simulink model "NLGuidance"  (R2016a)
settings: Solver=ode3  StartTime=0.0  StopTime=10.0  FixedStep=.02  RelTol=1e-3
model workspace (MAT data in the model file):
  F = [0.0104799567177; 0.0105274136759; 0.00258730184958; 0.00112291450915; 0.0065543125439; 0]
  N = 51
  S1 = [2.42464759278 -2.49697623385 -0.253883104432 -3.312058597 3.28063521535 2.42464759278 -2.49697623385 -0.253883104432 -3.312058597 3.28063521535 2.42464759278 -2.49697623385 ... (7515 elements, 5x1503)]
  S2 = [-47.5753524072 -52.4969762338 -50.2538831044 -53.312058597 -46.7193647847 -53.1933464928 -58.0206597562 -53.298625948 -53.0732596071 -45.5277132009 -58.8093605499 -63.5421671216 ... (7515 elements, 5x1503)]
  S3 = [-5.62481372887 -5.52769980874 -3.05143765206 0.237149289911 1.1849461568 -5.61799408553 -5.52368352234 -3.04474284358 0.238798989919 1.19165158379 -5.61601405716 -5.52150736543 ... (7515 elements, 5x1503)]
  S4 = [0 0 0 0 0 0 0 0 0 0 0 0 ... (7515 elements, 5x1503)]
  Vt = [0 0 0 0 0 0 0 0 0 0 0 0 ... (1503 elements, 501x3)]
  Vv = [1.1849461568 1.19165158379 1.19363427504 1.1947051518 1.20742767257 1.21177592763 1.21717805586 1.22205358332 1.22753574851 1.22892415591 1.22911717004 1.25058652202 ... (1503 elements, 501x3)]
  Vvmag = [6.45855507903 6.44973720458 6.44685088198 6.4408859639 6.4366826743 6.42659096353 6.42411891458 6.41278379056 6.40944425236 6.4051659263 6.38964384833 6.38667032718 ... (501 elements, 501x1)]
  X = [2.42464759278 -2.49697623385 -0.253883104432 -3.312058597 3.28063521535 -3.6978315289 -3.58806283515 -3.26410626081 1.58732884776 1.68742830515 1.89810778603 -3.58806283515 ... (72 elements, 6x12)]
  Xap1 = [3.53742766553 3.54841812521 3.55649436401 3.56301032299 3.56900127601 3.57285766144 3.57579889741 3.57816116305 3.57954580685 3.57954139291 3.5792899619 3.58161806007 ... (1503 elements, 501x3)]
  Xap2 = [3.00894026262 2.99947384008 2.99278206158 2.98751350515 2.98264302934 2.97978827516 2.97774180284 2.97617755456 2.97550435147 2.97614326838 2.97696071264 2.97513994677 ... (1503 elements, 501x3)]
  Xr = [10 11.2284720857 12.4539847001 13.6735561742 14.8879723634 16.0937793652 17.2959786101 18.4820399899 19.6645679603 20.8393619799 21.9947001613 23.1446286766 ... (1503 elements, 501x3)]
  Xrmag = [15.65732221 23.8105907731 30.9856356907 38.4540834067 46.0738528973 53.7662892745 61.5065103501 69.2725920166 77.0607192366 84.8582850512 92.6527324163 100.450411961 ... (501 elements, 501x1)]
  Xtarg = [3.28063521535 3.28063521535 3.28063521535 3.28063521535 3.28063521535 3.28063521535 3.28063521535 3.28063521535 3.28063521535 3.28063521535 3.28063521535 3.28063521535 ... (1503 elements, 501x3)]
  Xv = [-46.7193647847 -45.5277132009 -44.3340789258 -43.139373774 -41.9319461015 -40.7201701738 -39.502992118 -38.2809385346 -37.0534027861 -35.8244786302 -34.5953614602 -33.3447749382 ... (1503 elements, 501x3)]
  ans = [0  0  0; 2  2  2; 4  4  4]
  MCOS : class17 (value not decoded)
  cmd1 = []
  cmd2 = []
  count = 136
  curPath = '/Users/khouloud.gaaloul/Documents/Projects/QRA-Search/Problems/SimulinkTesting'
  MCOS : class17 (value not decoded)
  MCOS : class17 (value not decoded)
  MCOS : class17 (value not decoded)
  MCOS : class17 (value not decoded)
  d = 10
  dev = [0.998411888767 0.99782484185 0.997422855714 0.997059153759 0.99673360256 0.996441028681 0.996174188817 0.995929724086 0.995704685947 0.995496539497 0.995301805204 0.995118534567 ... (501 elements, 501x1)]
  diff = [-0.0110961446926 -0.0111456874882 -0.0111717248678 -0.0112203324043 -0.0112177067868 -0.0112470382447 -0.0112585651595 -0.0112536842015 -0.0112567920009 -0.0112598719834 -0.0112758132864 -0.011238461177 ... (500 elements, 500x1)]
  MCOS : class17 (value not decoded)
  MCOS : class17 (value not decoded)
  MCOS : class17 (value not decoded)
  handle : class17 (value not decoded)
  i = 26
  inputSize = 6
  j = 3
  list : struct (value not decoded)
  m = [-0.999723895919 -0.999364400237 -0.991672916331 -0.981758345493 -0.98121871348 -0.980992634152 -0.979214833695 -0.97816820181 -0.975813767607 -0.973821424379 -0.973796463479 -0.972935922229 ... (3006 elements, 1002x3)]
  modelpath = '/Users/khouloud.gaaloul/Documents/Projects/QRA-Search/SimulinkModels/4_nlguide/'
  mt = [0.997620134247 0.997296649802 0.994217918569 0.993324313281 0.991703646703 0.985900322398 0.985631450718 0.976402580538 0.973784078633 0.970318825583 0.969896216991 0.965968068121 ... (1503 elements, 501x3)]
  mv = [-0.993370609414 -0.990984924743 -0.989879999798 -0.982454455416 -0.979488128766 -0.978091228792 -0.976254482971 -0.973907633905 -0.96148789861 -0.959724271782 -0.942427931753 -0.941335472094 ... (1503 elements, 501x3)]
  n = 6
  nbrInputs = 4
  nbrTimeSteps = 501
  r2 = 1000000
  s = 4
  MCOS : class17 (value not decoded)
  sumOut = 1.13428583934e-06
  sumVl = 16.4352757808
  t = 501
  var : struct (value not decoded)
  varout : struct (value not decoded)
  x = [2.7049904163 8.31847210292 14.0416550116 19.9218605512 25.7958831948 31.6629046774 37.5137196427 43.3342242648 49.1594101201 54.9752404562 60.7952146721 66.6155429658 ... (501 elements, 501x1)]
  xo = [3.00894026262 2.99947384008 2.99278206158 2.98751350515 2.98264302934 2.97978827516 2.97774180284 2.97617755456 2.97550435147 2.97614326838 2.97696071264 2.97513994677 ... (501 elements, 501x1)]
  xt = [3.28063521535 3.28063521535 3.28063521535 3.28063521535 3.28063521535 3.28063521535 3.28063521535 3.28063521535 3.28063521535 3.28063521535 3.28063521535 3.28063521535 ... (501 elements, 501x1)]
  xv = [-46.7193647847 -45.5277132009 -44.3340789258 -43.139373774 -41.9319461015 -40.7201701738 -39.502992118 -38.2809385346 -37.0534027861 -35.8244786302 -34.5953614602 -33.3447749382 ... (501 elements, 501x1)]
  y = [3.6883959876 9.17834089576 14.9294898906 19.9030920073 24.7285315288 29.5033134454 34.2547577046 38.9972499457 43.7096979702 48.4166380479 53.1197368616 57.8142423866 ... (501 elements, 501x1)]
  yo = [2.64835074056 2.63493178346 2.62207989272 2.61010927833 2.59912240045 2.58878484686 2.57921418375 2.57035768583 2.56215199533 2.55453681534 2.54751560237 2.54111946622 ... (501 elements, 501x1)]
  yout = [3.00894026262 2.99947384008 2.99278206158 2.98751350515 2.98264302934 2.97978827516 2.97774180284 2.97617755456 2.97550435147 2.97614326838 2.97696071264 2.97513994677 ... (1503 elements, 501x3)]
  yt = [1.89810778603 1.89810778603 1.89810778603 1.89810778603 1.89810778603 1.89810778603 1.89810778603 1.89810778603 1.89810778603 1.89810778603 1.89810778603 1.89810778603 ... (501 elements, 501x1)]
  yv = [-48.101892214 -52.3846332875 -56.663611085 -60.93703548 -65.20593249 -69.4668713892 -73.7274049649 -77.9871267457 -82.2407780144 -86.4920761433 -90.7431651505 -94.9853167819 ... (501 elements, 501x1)]
  z = [4.49604856588 6.72999883369 12.0965927953 17.1688972661 22.1258781778 27.0326381497 31.9068218628 36.7791547029 41.639146818 46.4962544595 51.3440742559 56.1827474075 ... (501 elements, 501x1)]
  zo = [4.92497802224 4.93706839336 4.94912096266 4.96029006041 4.97012356487 4.97983400233 4.98881546471 4.99704254051 5.00481819698 5.01242680713 5.01939367699 5.02450802519 ... (501 elements, 501x1)]
  zt = [4.32221989343 4.32221989343 4.32221989343 4.32221989343 4.32221989343 4.32221989343 4.32221989343 4.32221989343 4.32221989343 4.32221989343 4.32221989343 4.32221989343 ... (501 elements, 501x1)]
  zv = [45.6777801066 48.680795879 51.6837683233 54.6803231469 57.6757020576 60.666276224 63.6537597154 66.6335569064 69.6091973174 72.5839099026 75.5526555129 78.520090746 ... (501 elements, 501x1)]
(part 2 of 2)

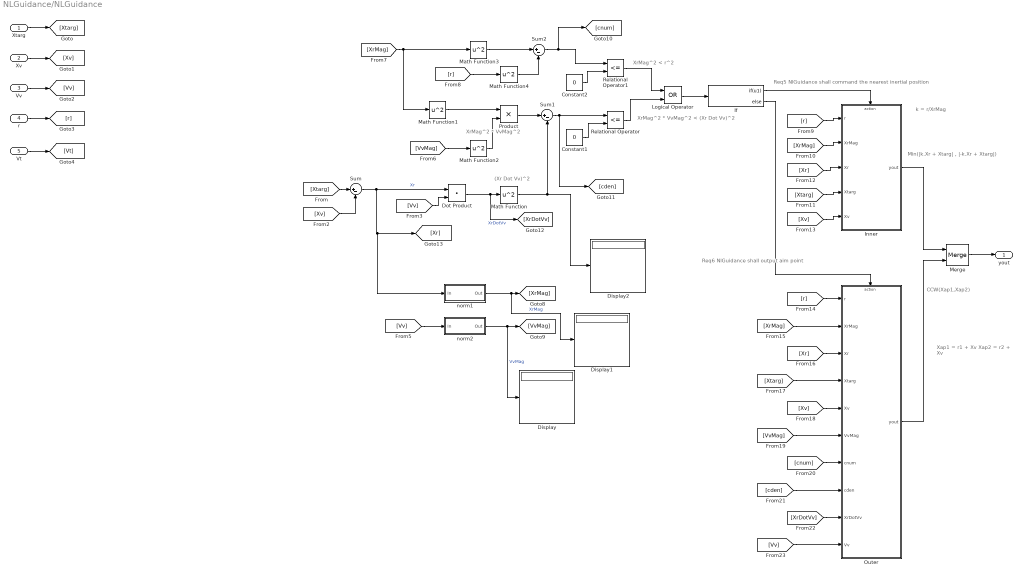
== system NLGuidance/NLGuidance ==
  note: XrMag^2 < r^2
  note: Req5 NlGuidance shall command the nearest inertial position
  note: XrMag^2 * VvMag^2
  note: (Xr Dot Vv)^2
  note: XrMag^2 * VvMag^2 < (Xr Dot Vv)^2
  note: k = r/XrMag
  note: Min(|k.Xr + Xtarg| , |-k.Xr + Xtarg|)
  note: Xap1 = r1 + Xv
      | Xap2 = r2 + Xv
  note: CCW(Xap1,Xap2)
  note: Req6 NlGuidance shall output aim point
  Xtarg : Inport
  Xv : Inport  Port=2
  Vv : Inport  Port=3
  r : Inport  Port=4
  Vt : Inport  Port=5
  Constant1 : Constant  Value=0
  Constant2 : Constant  Value=0
  Display : Display
  Display1 : Display
  Display2 : Display
  Dot Product : DotProduct  InputSameDT=on  OutDataTypeStr=Inherit: Inherit via internal rule
  If : If  IfExpression=u1
  Inner : Subsystem
  Logical Operator : Logic  Operator=OR  AllPortsSameDT=off  OutDataTypeStr=boolean
  Math Function{,1..4} (5 alike) : Math  Operator=square  SaturateOnIntegerOverflow=on
  Merge : Merge
  Outer : Subsystem
  Product : Product  RndMeth=Zero
  Relational Operator : RelationalOperator  Operator=<=  OutDataTypeStr=boolean
  Relational Operator1 : RelationalOperator  Operator=<=  OutDataTypeStr=boolean
  Sum : Sum  Inputs=|+-
  Sum1 : Sum  Inputs=|+-
  Sum2 : Sum  Inputs=|+-
  norm1 : Subsystem
  norm2 : Subsystem
  yout : Outport
  wires:
  Xtarg/1 -> [Xtarg]
  Xv/1 -> [Xv]
  Vv/1 -> [Vv]
  r/1 -> [r]
  Vt/1 -> [Vt]
  [Xtarg] -> Sum/1
  [Xv] -> Sum/2
  Sum/1 -> norm1/1(In), [Xr], Dot Product/1  "Xr"
  [Vv] -> Dot Product/2
  Dot Product/1 -> [XrDotVv], Math Function/1  "XrDotVv"
  norm1/1(Out) -> Display1/1, [XrMag]  "XrMag"
  [Vv] -> norm2/1(In)
  norm2/1(Out) -> Display/1, [VvMag]  "VvMag"
  Math Function/1 -> Display2/1, Sum1/2
  [VvMag] -> Math Function2/1
  Math Function1/1 -> Product/1
  Math Function2/1 -> Product/2
  Product/1 -> Sum1/1
  Sum1/1 -> [cden], Relational Operator/1
  Constant1/1 -> Relational Operator/2
  Relational Operator/1 -> Logical Operator/2
  Sum2/1 -> [cnum], Relational Operator1/1
  Constant2/1 -> Relational Operator1/2
  Relational Operator1/1 -> Logical Operator/1
  Math Function3/1 -> Sum2/1
  [XrMag] -> Math Function1/1, Math Function3/1
  Math Function4/1 -> Sum2/2
  [r] -> Math Function4/1
  [r] -> Inner/1(r)
  [XrMag] -> Inner/2(XrMag)
  Logical Operator/1 -> If/1
  [Xtarg] -> Inner/4(Xtarg)
  [Xr] -> Inner/3(Xr)
  [Xv] -> Inner/5(Xv)
  Inner/1(yout) -> Merge/1
  Outer/1(yout) -> Merge/2
  If/1 -> Inner/Action
  If/2 -> Outer/Action
  [r] -> Outer/1(r)
  [XrMag] -> Outer/2(XrMag)
  [Xr] -> Outer/3(Xr)
  [Xtarg] -> Outer/4(Xtarg)
  [Xv] -> Outer/5(Xv)
  [VvMag] -> Outer/6(VvMag)
  [cnum] -> Outer/7(cnum)
  [cden] -> Outer/8(cden)
  [XrDotVv] -> Outer/9(XrDotVv)
  [Vv] -> Outer/10(Vv)
  Merge/1 -> yout/1

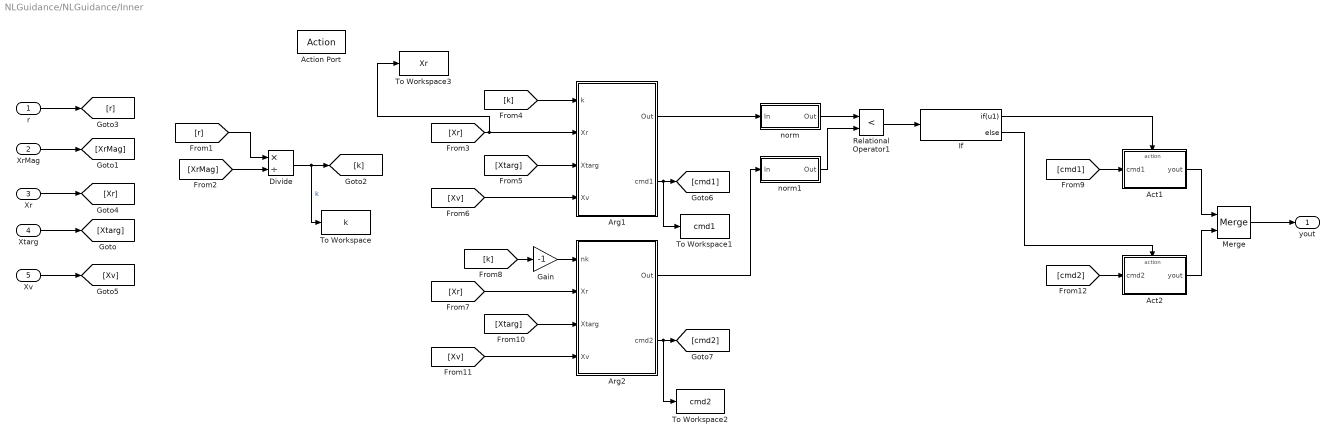
== system NLGuidance/NLGuidance/Inner ==
  r : Inport
  XrMag : Inport  Port=2
  Xr : Inport  Port=3
  Xtarg : Inport  Port=4
  Xv : Inport  Port=5
  Action Port : ActionPort  ActionType=then
  Act1 : Subsystem
  Act2 : Subsystem
  Arg1 : Subsystem
  Arg2 : Subsystem
  Divide : Product  Inputs=*/
  Gain : Gain  Gain=-1
  If : If  IfExpression=u1
  Merge : Merge
  Relational Operator1 : RelationalOperator  Operator=<  OutDataTypeStr=boolean
  To Workspace : ToWorkspace  VariableName=k  SaveFormat=Timeseries  SampleTime=-1
  To Workspace1 : ToWorkspace  VariableName=cmd1  SampleTime=-1
  To Workspace2 : ToWorkspace  VariableName=cmd2  SampleTime=-1
  To Workspace3 : ToWorkspace  VariableName=Xr  SaveFormat=Timeseries  SampleTime=-1
  norm : Subsystem
  norm1 : Subsystem
  yout : Outport
  wires:
  Divide/1 -> To Workspace/1, [k]  "k"
  r/1 -> [r]
  XrMag/1 -> [XrMag]
  Xtarg/1 -> [Xtarg]
  [r] -> Divide/1
  [XrMag] -> Divide/2
  Xr/1 -> [Xr]
  Xv/1 -> [Xv]
  norm/1(Out) -> Relational Operator1/1
  norm1/1(Out) -> Relational Operator1/2
  Arg1/1(Out) -> norm/1(In)
  [k] -> Arg1/1(k)
  [Xr] -> To Workspace3/1, Arg1/2(Xr)
  [Xtarg] -> Arg1/3(Xtarg)
  [Xv] -> Arg1/4(Xv)
  Relational Operator1/1 -> If/1
  [Xr] -> Arg2/2(Xr)
  [Xtarg] -> Arg2/3(Xtarg)
  [Xv] -> Arg2/4(Xv)
  Arg2/1(Out) -> norm1/1(In)
  [k] -> Gain/1
  Gain/1 -> Arg2/1(nk)
  Arg1/2(cmd1) -> To Workspace1/1, [cmd1]
  Arg2/2(cmd2) -> To Workspace2/1, [cmd2]
  [cmd1] -> Act1/1(cmd1)
  [cmd2] -> Act2/1(cmd2)
  Act1/1(yout) -> Merge/1
  Act2/1(yout) -> Merge/2
  Merge/1 -> yout/1
  If/1 -> Act1/Action
  If/2 -> Act2/Action

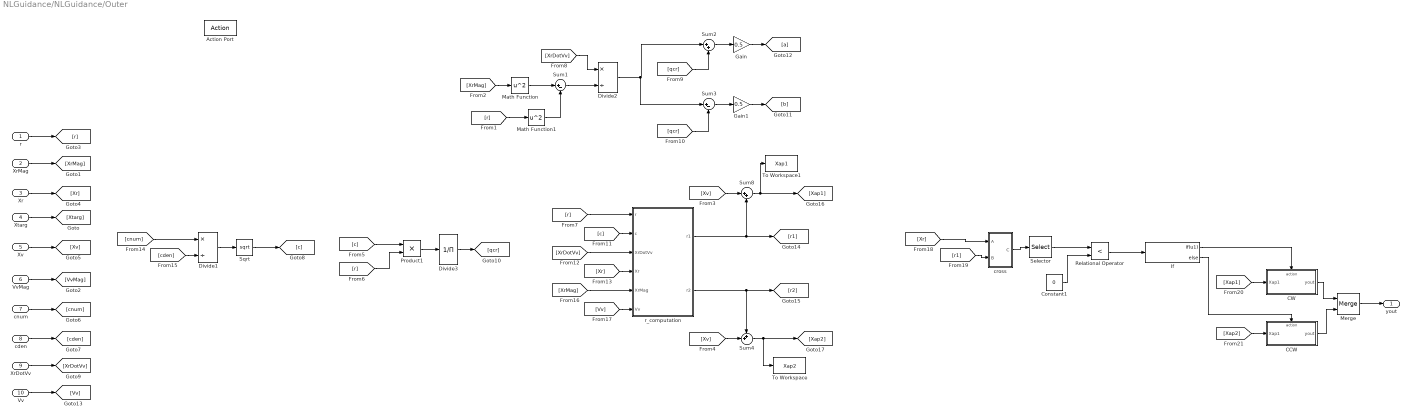
== system NLGuidance/NLGuidance/Outer ==
  r : Inport
  XrMag : Inport  Port=2
  Xr : Inport  Port=3
  Xtarg : Inport  Port=4
  Xv : Inport  Port=5
  VvMag : Inport  Port=6
  cnum : Inport  Port=7
  cden : Inport  Port=8
  XrDotVv : Inport  Port=9
  Vv : Inport  Port=10
  Action Port : ActionPort  ActionType=else
  CCW : Subsystem
  CW : Subsystem
  Constant1 : Constant  Value=0
  Divide1 : Product  Inputs=*/
  Divide2 : Product  Inputs=*/
  Divide3 : Product  Inputs=/
  Gain : Gain  Gain=0.5
  Gain1 : Gain  Gain=0.5
  If : If  IfExpression=u1
  Math Function : Math  Operator=square  SaturateOnIntegerOverflow=on
  Math Function1 : Math  Operator=square  SaturateOnIntegerOverflow=on
  Merge : Merge
  Product1 : Product
  Relational Operator : RelationalOperator  Operator=<  OutDataTypeStr=boolean
  Selector : Selector  InputPortWidth=3  IndexOptions=Index vector (dialog)  Indices=[3]  OutputSizes=1
  Sqrt : Sqrt  SaturateOnIntegerOverflow=on
  Sum1 : Sum  Inputs=|+-
  Sum2 : Sum  Inputs=|++
  Sum3 : Sum  Inputs=|+-
  Sum4 : Sum  Inputs=++|
  Sum8 : Sum  Inputs=|++
  To Workspace : ToWorkspace  VariableName=Xap2  SampleTime=-1
  To Workspace1 : ToWorkspace  VariableName=Xap1  SampleTime=-1
  cross : Subsystem
  r_computation : Subsystem
  yout : Outport
  wires:
  r/1 -> [r]
  XrMag/1 -> [XrMag]
  Xtarg/1 -> [Xtarg]
  Xr/1 -> [Xr]
  Xv/1 -> [Xv]
  [XrMag] -> Math Function/1
  [r] -> Math Function1/1
  VvMag/1 -> [VvMag]
  cnum/1 -> [cnum]
  [cnum] -> Divide1/1
  [cden] -> Divide1/2
  Divide1/1 -> Sqrt/1
  Sqrt/1 -> [c]
  cden/1 -> [cden]
  XrDotVv/1 -> [XrDotVv]
  [c] -> Product1/1
  [r] -> Product1/2
  Math Function/1 -> Sum1/1
  Math Function1/1 -> Sum1/2
  Sum1/1 -> Divide2/2
  [XrDotVv] -> Divide2/1
  Divide2/1 -> Sum3/1, Sum2/1
  Sum2/1 -> Gain/1
  Sum3/1 -> Gain1/1
  Product1/1 -> Divide3/1
  Divide3/1 -> [qcr]
  [qcr] -> Sum2/2
  [qcr] -> Sum3/2
  Gain1/1 -> [b]
  Gain/1 -> [a]
  Vv/1 -> [Vv]
  r_computation/1(r1) -> Sum8/2, [r1]
  r_computation/2(r2) -> Sum4/1, [r2]
  [Xv] -> Sum8/1
  [Xv] -> Sum4/2
  Sum4/1 -> To Workspace/1, [Xap2]
  [r] -> r_computation/1(r)
  [c] -> r_computation/2(c)
  [XrDotVv] -> r_computation/3(XrDotVv)
  [Xr] -> r_computation/4(Xr)
  [XrMag] -> r_computation/5(XrMag)
  [Vv] -> r_computation/6(Vv)
  cross/1(C) -> Selector/1
  [Xr] -> cross/1(A)
  [r1] -> cross/2(B)
  Constant1/1 -> Relational Operator/2
  Selector/1 -> Relational Operator/1
  Relational Operator/1 -> If/1
  If/1 -> CW/Action
  [Xap1] -> CW/1(Xap1)
  If/2 -> CCW/Action
  [Xap2] -> CCW/1(Xap1)
  CW/1(yout) -> Merge/1
  CCW/1(yout) -> Merge/2
  Merge/1 -> yout/1
  Sum8/1 -> To Workspace1/1, [Xap1]

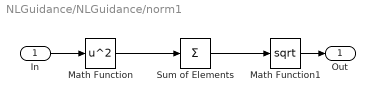
== system NLGuidance/NLGuidance/norm1 ==
  In : Inport
  Math Function : Math  Operator=square  SaturateOnIntegerOverflow=on
  Math Function1 : Math  Operator=sqrt  SaturateOnIntegerOverflow=on
  Sum of Elements : Sum  Inputs=+
  Out : Outport
  wires:
  Math Function/1 -> Sum of Elements/1
  Sum of Elements/1 -> Math Function1/1
  In/1 -> Math Function/1
  Math Function1/1 -> Out/1

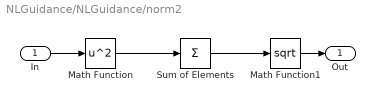
== system NLGuidance/NLGuidance/norm2 ==
  In : Inport
  Math Function : Math  Operator=square  SaturateOnIntegerOverflow=on
  Math Function1 : Math  Operator=sqrt  SaturateOnIntegerOverflow=on
  Sum of Elements : Sum  Inputs=+
  Out : Outport
  wires:
  Math Function1/1 -> Out/1
  In/1 -> Math Function/1
  Sum of Elements/1 -> Math Function1/1
  Math Function/1 -> Sum of Elements/1

== system NLGuidance/NLGuidance/Inner/Act1 ==
  cmd1 : Inport
  Action Port : ActionPort  ActionType=then
  yout : Outport
  wires:
  cmd1/1 -> yout/1

== system NLGuidance/NLGuidance/Inner/Act2 ==
  cmd2 : Inport
  Action Port : ActionPort  ActionType=else
  yout : Outport
  wires:
  cmd2/1 -> yout/1

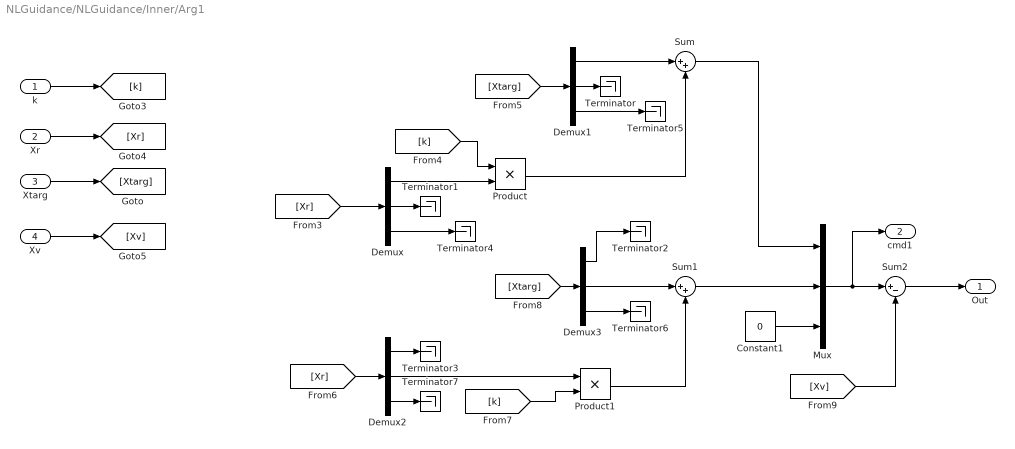
== system NLGuidance/NLGuidance/Inner/Arg1 ==
  k : Inport
  Xr : Inport  Port=2
  Xtarg : Inport  Port=3
  Xv : Inport  Port=4
  Constant1 : Constant  Value=0
  Demux{,1..3} (4 alike) : Demux  Outputs=3
  Mux : Mux  Inputs=3
  Product : Product  RndMeth=Zero
  Product1 : Product  RndMeth=Zero
  Sum : Sum  Inputs=|++
  Sum1 : Sum  Inputs=|++
  Sum2 : Sum  Inputs=|+-
  Terminator{,1..7} (8 alike) : Terminator
  Out : Outport
  cmd1 : Outport  Port=2
  wires:
  Mux/1 -> cmd1/1, Sum2/1
  Demux3/3 -> Terminator6/1
  Demux/2 -> Terminator1/1
  [Xr] -> Demux2/1
  Sum/1 -> Mux/1
  Demux1/2 -> Terminator/1
  [k] -> Product1/2
  Constant1/1 -> Mux/3
  Demux3/2 -> Sum1/1
  Demux2/1 -> Terminator3/1
  [Xtarg] -> Demux1/1
  Product/1 -> Sum/2
  [k] -> Product/1
  Demux/1 -> Product/2
  [Xr] -> Demux/1
  Sum1/1 -> Mux/2
  Demux1/1 -> Sum/1
  Demux2/3 -> Terminator7/1
  [Xtarg] -> Demux3/1
  Sum2/1 -> Out/1
  Demux/3 -> Terminator4/1
  [Xv] -> Sum2/2
  Demux3/1 -> Terminator2/1
  Demux2/2 -> Product1/1
  Product1/1 -> Sum1/2
  Demux1/3 -> Terminator5/1
  k/1 -> [k]
  Xtarg/1 -> [Xtarg]
  Xr/1 -> [Xr]
  Xv/1 -> [Xv]

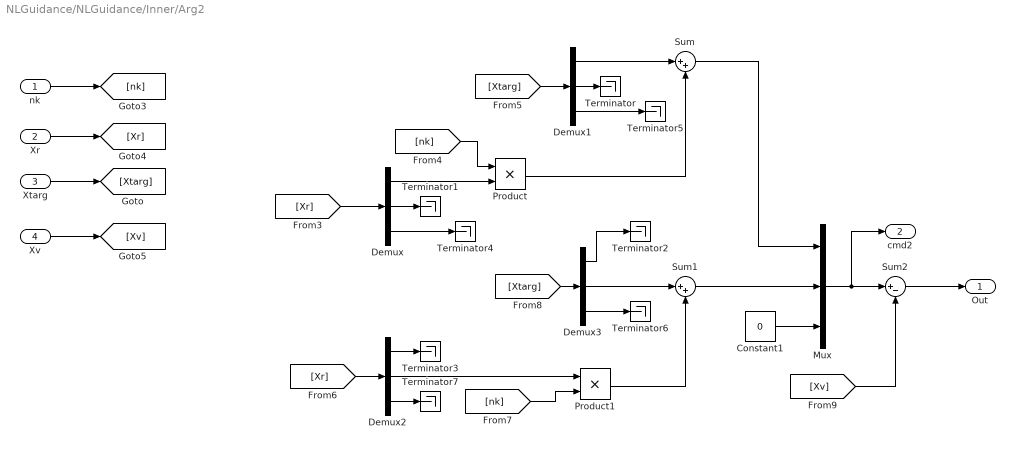
== system NLGuidance/NLGuidance/Inner/Arg2 ==
  nk : Inport
  Xr : Inport  Port=2
  Xtarg : Inport  Port=3
  Xv : Inport  Port=4
  Constant1 : Constant  Value=0
  Demux{,1..3} (4 alike) : Demux  Outputs=3
  Mux : Mux  Inputs=3
  Product : Product  RndMeth=Zero
  Product1 : Product  RndMeth=Zero
  Sum : Sum  Inputs=|++
  Sum1 : Sum  Inputs=|++
  Sum2 : Sum  Inputs=|+-
  Terminator{,1..7} (8 alike) : Terminator
  Out : Outport
  cmd2 : Outport  Port=2
  wires:
  Xv/1 -> [Xv]
  Xr/1 -> [Xr]
  Xtarg/1 -> [Xtarg]
  nk/1 -> [nk]
  Demux1/3 -> Terminator5/1
  Product1/1 -> Sum1/2
  Demux2/2 -> Product1/1
  Demux3/1 -> Terminator2/1
  [Xv] -> Sum2/2
  Demux/3 -> Terminator4/1
  Sum2/1 -> Out/1
  [Xtarg] -> Demux3/1
  Demux2/3 -> Terminator7/1
  Demux1/1 -> Sum/1
  Sum1/1 -> Mux/2
  [Xr] -> Demux/1
  Demux/1 -> Product/2
  [nk] -> Product/1
  Product/1 -> Sum/2
  [Xtarg] -> Demux1/1
  Demux2/1 -> Terminator3/1
  Demux3/2 -> Sum1/1
  Constant1/1 -> Mux/3
  [nk] -> Product1/2
  Demux1/2 -> Terminator/1
  Sum/1 -> Mux/1
  [Xr] -> Demux2/1
  Demux/2 -> Terminator1/1
  Demux3/3 -> Terminator6/1
  Mux/1 -> cmd2/1, Sum2/1

== system NLGuidance/NLGuidance/Inner/norm ==
  In : Inport
  Math Function : Math  Operator=square  SaturateOnIntegerOverflow=on
  Math Function1 : Math  Operator=sqrt  SaturateOnIntegerOverflow=on
  Sum of Elements : Sum  Inputs=+
  Out : Outport
  wires:
  Math Function1/1 -> Out/1
  In/1 -> Math Function/1
  Sum of Elements/1 -> Math Function1/1
  Math Function/1 -> Sum of Elements/1

== system NLGuidance/NLGuidance/Inner/norm1 ==
  In : Inport
  Math Function : Math  Operator=square  SaturateOnIntegerOverflow=on
  Math Function1 : Math  Operator=sqrt  SaturateOnIntegerOverflow=on
  Sum of Elements : Sum  Inputs=+
  Out : Outport
  wires:
  Math Function/1 -> Sum of Elements/1
  Sum of Elements/1 -> Math Function1/1
  In/1 -> Math Function/1
  Math Function1/1 -> Out/1

== system NLGuidance/NLGuidance/Outer/CCW ==
  Xap1 : Inport
  Action Port : ActionPort  ActionType=else
  yout : Outport
  wires:
  Xap1/1 -> yout/1

== system NLGuidance/NLGuidance/Outer/CW ==
  Xap1 : Inport
  Action Port : ActionPort  ActionType=then
  yout : Outport
  wires:
  Xap1/1 -> yout/1

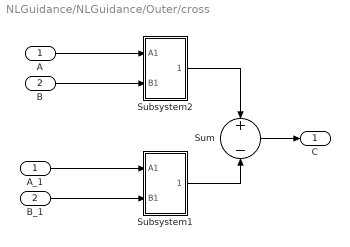
== system NLGuidance/NLGuidance/Outer/cross ==
  A : Inport
  B : Inport  Port=2
  A_1 : InportShadow
  B_1 : InportShadow  Port=2
  Subsystem1 : Subsystem
  Subsystem2 : Subsystem
  Sum : Sum  Inputs=+|-  SaturateOnIntegerOverflow=on  InputSameDT=on  OutDataTypeStr=Inherit: Same as first input
  C : Outport
  wires:
  B/1 -> Subsystem2/2(B1)
  A_1/1 -> Subsystem1/1(A1)
  A/1 -> Subsystem2/1(A1)
  Subsystem2/1(Out1) -> Sum/1
  B_1/1 -> Subsystem1/2(B1)
  Sum/1 -> C/1
  Subsystem1/1(Out1) -> Sum/2

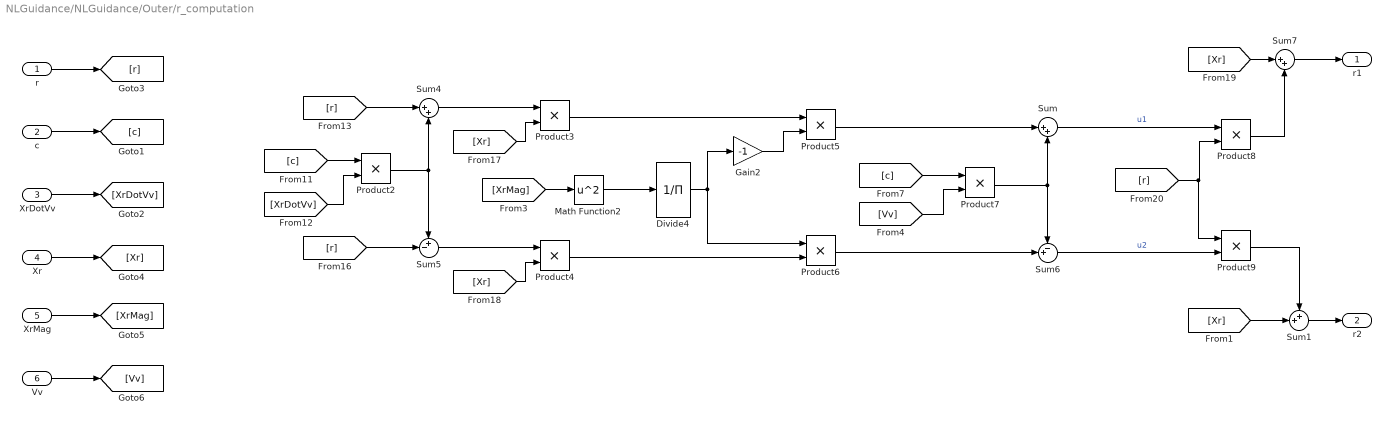
== system NLGuidance/NLGuidance/Outer/r_computation ==
  r : Inport
  c : Inport  Port=2
  XrDotVv : Inport  Port=3
  Xr : Inport  Port=4
  XrMag : Inport  Port=5
  Vv : Inport  Port=6
  Divide4 : Product  Inputs=/
  Gain2 : Gain  Gain=-1
  Math Function2 : Math  Operator=square  SaturateOnIntegerOverflow=on
  Product{2..9} (8 alike) : Product
  Sum : Sum  Inputs=|++
  Sum1 : Sum  Inputs=++|
  Sum4 : Sum  Inputs=|++
  Sum5 : Sum  Inputs=+-|
  Sum6 : Sum  Inputs=-+|
  Sum7 : Sum  Inputs=|++
  r1 : Outport
  r2 : Outport  Port=2
  wires:
  [r] -> Sum4/1
  Sum6/1 -> Product9/2  "u2"
  Gain2/1 -> Product5/2
  Product4/1 -> Product6/2
  [XrDotVv] -> Product2/2
  [Xr] -> Product4/2
  Product3/1 -> Product5/1
  Divide4/1 -> Product6/1, Gain2/1
  Sum5/1 -> Product4/1
  [Xr] -> Sum7/1
  [Vv] -> Product7/2
  Product7/1 -> Sum/2, Sum6/1
  [r] -> Product9/1, Product8/2
  Product8/1 -> Sum7/2
  Sum7/1 -> r1/1
  Product6/1 -> Sum6/2
  Product5/1 -> Sum/1
  [Xr] -> Product3/2
  [c] -> Product7/1
  Math Function2/1 -> Divide4/1
  [XrMag] -> Math Function2/1
  [c] -> Product2/1
  Sum4/1 -> Product3/1
  Sum/1 -> Product8/1  "u1"
  Product2/1 -> Sum5/1, Sum4/2
  [r] -> Sum5/2
  r/1 -> [r]
  c/1 -> [c]
  XrDotVv/1 -> [XrDotVv]
  Xr/1 -> [Xr]
  XrMag/1 -> [XrMag]
  Vv/1 -> [Vv]
  Product9/1 -> Sum1/1
  [Xr] -> Sum1/2
  Sum1/1 -> r2/1

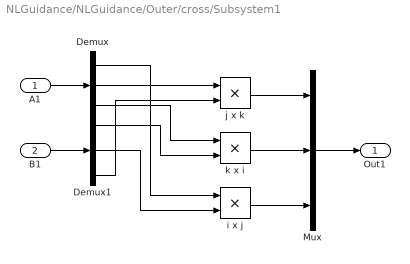
== system NLGuidance/NLGuidance/Outer/cross/Subsystem1 ==
  A1 : Inport
  B1 : Inport  Port=2
  Demux : Demux  Outputs=3
  Demux1 : Demux  Outputs=3
  Mux : Mux  Inputs=3
  i x j : Product  SaturateOnIntegerOverflow=on  InputSameDT=on  OutDataTypeStr=Inherit: Same as first input
  j x k : Product  SaturateOnIntegerOverflow=on  InputSameDT=on  OutDataTypeStr=Inherit: Same as first input
  k x i : Product  SaturateOnIntegerOverflow=on  InputSameDT=on  OutDataTypeStr=Inherit: Same as first input
  Out1 : Outport
  wires:
  Demux/2 -> j x k/1
  Demux1/3 -> j x k/2
  A1/1 -> Demux/1
  Demux/3 -> k x i/1
  Mux/1 -> Out1/1
  j x k/1 -> Mux/1
  B1/1 -> Demux1/1
  k x i/1 -> Mux/2
  Demux1/2 -> i x j/2
  i x j/1 -> Mux/3
  Demux/1 -> i x j/1
  Demux1/1 -> k x i/2

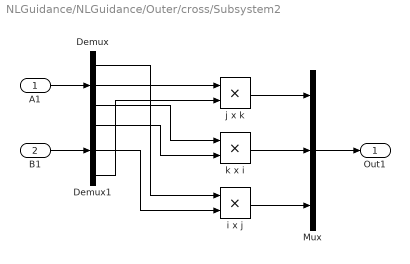
== system NLGuidance/NLGuidance/Outer/cross/Subsystem2 ==
  A1 : Inport
  B1 : Inport  Port=2
  Demux : Demux  Outputs=3
  Demux1 : Demux  Outputs=3
  Mux : Mux  Inputs=3
  i x j : Product  SaturateOnIntegerOverflow=on  InputSameDT=on  OutDataTypeStr=Inherit: Same as first input
  j x k : Product  SaturateOnIntegerOverflow=on  InputSameDT=on  OutDataTypeStr=Inherit: Same as first input
  k x i : Product  SaturateOnIntegerOverflow=on  InputSameDT=on  OutDataTypeStr=Inherit: Same as first input
  Out1 : Outport
  wires:
  Demux1/1 -> k x i/2
  Demux/1 -> i x j/1
  i x j/1 -> Mux/3
  Demux1/2 -> i x j/2
  k x i/1 -> Mux/2
  B1/1 -> Demux1/1
  j x k/1 -> Mux/1
  Mux/1 -> Out1/1
  Demux/3 -> k x i/1
  A1/1 -> Demux/1
  Demux1/3 -> j x k/2
  Demux/2 -> j x k/1
